simulink model "LookupTableND_2D_spline"  (R2015a)
settings: Solver=FixedStepDiscrete  StartTime=0.0  StopTime=10.0  FixedStep=0.2  RelTol=1e-3
settings Model: Creator=hbourbou  LastModifiedBy=ktrinh
settings DataIOCC: SaveFormat=StructureWithTime
settings HardwareCC: ProdBitPerPointer=64  ProdLargestAtomicFloat=Float  ProdIntDivRoundTo=Zero  ProdEndianess=LittleEndian  ProdHWDeviceType=Specified
settings GRTTargetCC: GeneratePreprocessorConditionals=Use local settings

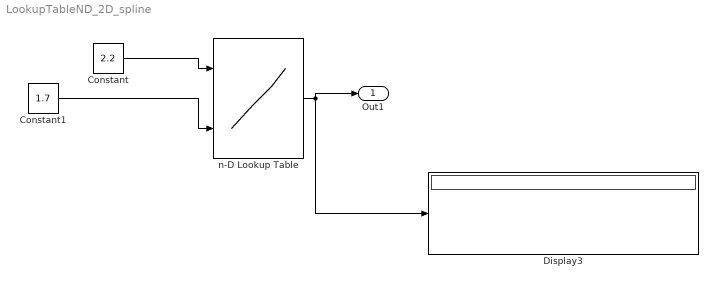
== system LookupTableND_2D_spline ==
  Constant : Constant  Value=2.2
  Constant1 : Constant  Value=1.7
  Display3 : Display
  n-D Lookup Table : Lookup_n-D  BreakpointsForDimension1=[1 2 3]  BreakpointsForDimension2=[0 1 2]  BreakpointsForDimension3=[5 6]  Table=[1 12 3; 14 5 6 ; 7 8 19]  InterpMethod=Cubic spline  InternalRulePriority=Speed  RndMeth=Simplest  InputSameDT=on
  Out1 : Outport
  wires:
  Constant/1 -> n-D Lookup Table/1
  Constant1/1 -> n-D Lookup Table/2
  n-D Lookup Table/1 -> Out1/1, Display3/1
